simulink model "exploded_cbd"  (R2025b)
settings: Solver=VariableStepAuto  StartTime=0.0  StopTime=10.0  RelTol=1e-3
PreLoadFcn:
  | load 'Control Block Diagram'\contact_force.mat
model workspace (MAT data in the model file):
  B_imp = 1
  INA125_gain = 604
  J_imp = 1
  K_d = 1
  K_f = 1
  K_i = 1
  K_imp = 1
  K_p = 1
  finger_length = 0.105
  full_ROM = 90
  joint_pulley_diam = 0.1
  sine_freq_Hz = 2
libraries: simulink x3
settings Model: Creator=Madeline  LastModifiedBy=Madeline

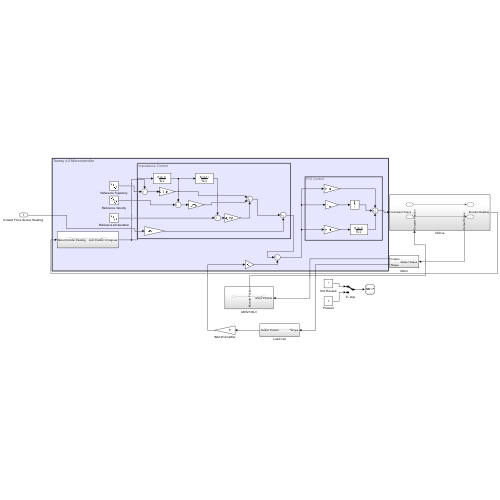
[thumbnail: Simulink's stored preview of the top-level diagram]
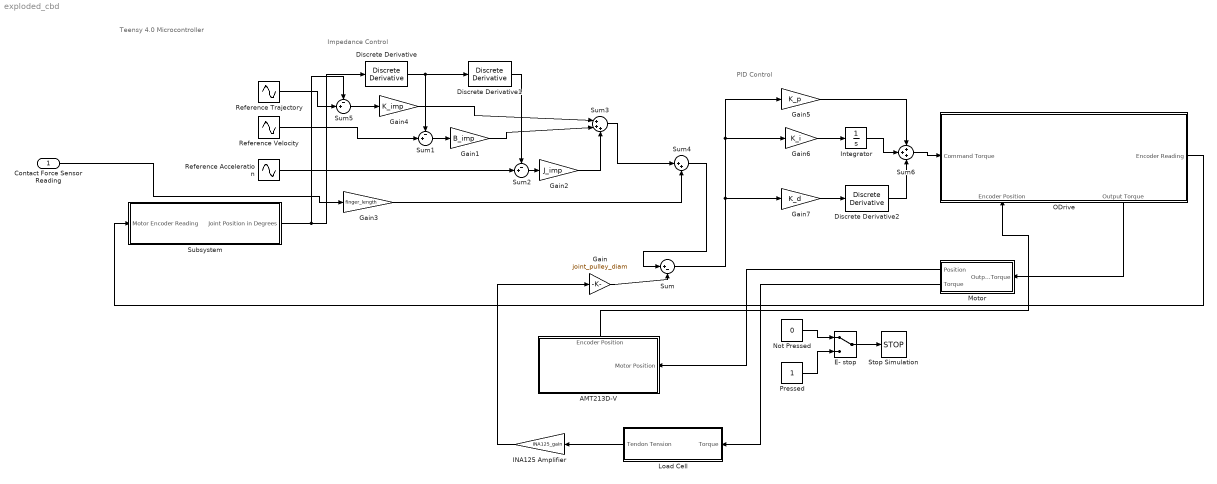
== system exploded_cbd ==
  note: PID Control
  note: Impedance Control
  note: Teensy 4.0 Microcontroller
  "Contact Force Sensor Reading " : Inport
  " E- stop" : ManualSwitch
  AMT213D-V : Subsystem
      settings: PortSchema="{\"entries\":[{\"content\":{\"sides\":[{\"content\":{\"connectorIds\":[\"In1\"]},\"type\":\"ConnectorPlacement.EquallySpacedRectSide\",\"uuid\":\"88afd67f-3209-48d2-80be-27a9c6027e98\"},{\"content\":{\"side\":\"RIGHT\"},\"type\":\"ConnectorPlacement.EquallySpacedRectSide\",\"uuid\":\"6bd83a64-80e2-4e6b-a2e1-60e2a1b1e7d1\"},{\"content\":{\"connectorIds\":[\"Out1\"],\"side\":\"TOP\"},\"type\":\"ConnectorPlacement.EquallySpacedRectSide\",\"uuid\":\"ca5e5761-7c4c-4ffd-94f8-cf864c9b5854\"}]},\"type\":\"ConnectorPlacement.EquallySpacedConnector\",\"uuid\":\"578619f2-0797-4ece-88f8-3f0e3f24fe58\"}],\"packageUris\":[\"http://schema.mathworks.com/mf0/Connector/R2020b\"],\"version\":\"1.0\"}"
  Discrete Derivative : simulink/Discrete/Discrete Derivative  gainval=1.0  ICPrevScaledInput=0.0  OutMin=[]  OutMax=[]  OutDataType=fixdt(1, 16)  OutScaling=2^-10  DoSatur=off
  Discrete Derivative1 : simulink/Discrete/Discrete Derivative  gainval=1.0  ICPrevScaledInput=0.0  OutMin=[]  OutMax=[]  OutDataType=fixdt(1, 16)  OutScaling=2^-10  DoSatur=off
  Discrete Derivative2 : simulink/Discrete/Discrete Derivative  gainval=1.0  ICPrevScaledInput=0.0  OutMin=[]  OutMax=[]  OutDataType=fixdt(1, 16)  OutScaling=2^-10  DoSatur=off
  Gain : Gain  Gain=joint_pulley_diam
  Gain1 : Gain  Gain=B_imp
  Gain2 : Gain  Gain=J_imp
  Gain3 : Gain  Gain=finger_length
  Gain4 : Gain  Gain=K_imp
  Gain5 : Gain  Gain=K_p
  Gain6 : Gain  Gain=K_i
  Gain7 : Gain  Gain=K_d
  INA125 Amplifier : Gain  Gain=INA125_gain
  Integrator : Integrator
  Load Cell : Subsystem
  Motor : Subsystem
  Not Pressed : Constant  Value=0
  ODrive : Subsystem
      settings: PortSchema="{\"entries\":[{\"content\":{\"sides\":[{\"content\":{\"connectorIds\":[\"In1\"]},\"type\":\"ConnectorPlacement.EquallySpacedRectSide\",\"uuid\":\"c97f3b25-cb08-4b77-804d-5691f1a52caa\"},{\"content\":{\"connectorIds\":[\"Out1\"],\"side\":\"RIGHT\"},\"type\":\"ConnectorPlacement.EquallySpacedRectSide\",\"uuid\":\"fc8ddf87-a458-4f73-a642-c7dd3d8cebff\"},{\"content\":{\"side\":\"TOP\"},\"type\":\"ConnectorPlacement.EquallySpacedRectSide\",\"uuid\":\"bec86457-f3cb-49fd-a085-c16f63c32d9e\"},{\"content\":{\"connectorIds\":[\"In2\",\"Out2\"],\"side\":\"BOTTOM\"},\"type\":\"ConnectorPlacement.EquallySpacedRectSide\",\"uuid\":\"4c0a5cbf-4f1d-4d43-a541-d1307432e3c9\"}]},\"type\":\"ConnectorPlacement.EquallySpacedConnector\",\"uuid\":\"94b3d347-19f8-405c-b5ff-c5a65504f3eb\"}],\"packageUris\":[\"http://schema.mathworks.com/mf0/Connector/R2020b\"],\"version\":\"1.0\"}"
  Pressed : Constant
  Reference Acceleration : Sin  Amplitude=-0.75*full_ROM*(sine_freq_Hz*2*pi)^2  Frequency=sine_freq_Hz*2*pi  SampleTime=0
  Reference Trajectory : Sin  Amplitude=0.75*full_ROM  Frequency=sine_freq_Hz*2*pi  SampleTime=0
  Reference Velocity : Sin  Amplitude=0.75*full_ROM*sine_freq_Hz*2*pi  Frequency=sine_freq_Hz*2*pi  Phase=pi/2  SampleTime=0
  Stop Simulation : Stop
  Subsystem : Subsystem
  Sum : Sum  Inputs=|+-
  Sum1 : Sum  Inputs=-+|
  Sum2 : Sum  Inputs=-+|
  Sum3 : Sum  Inputs=|+++
  Sum4 : Sum  Inputs=|++
  Sum5 : Sum  Inputs=-+|
  Sum6 : Sum  Inputs=+++
  wires:
  ODrive/2("Output Torque ") -> Motor/1("Output Torque ")
  Motor/1("Position ") -> AMT213D-V/1(Motor Position)
  Sum6/1 -> ODrive/1(Command Torque)
  AMT213D-V/1(Encoder Position) -> ODrive/2(Encoder Position)
  Motor/2(Torque) -> Load Cell/1(Torque)
  Not Pressed/1 -> " E- stop"/1
  Pressed/1 -> " E- stop"/2
  " E- stop"/1 -> Stop Simulation/1
  Load Cell/1(Tendon Tension) -> INA125 Amplifier/1
  Gain/1 -> Sum/2
  INA125 Amplifier/1 -> Gain/1
  Sum4/1 -> Sum/1
  ODrive/1(Encoder Reading) -> Subsystem/1(Motor Encoder Reading)
  Sum3/1 -> Sum4/1
  Gain3/1 -> Sum4/2
  "Contact Force Sensor Reading "/1 -> Gain3/1
  Gain2/1 -> Sum3/3
  Gain1/1 -> Sum3/2
  Gain4/1 -> Sum3/1
  Sum2/1 -> Gain2/1
  Sum1/1 -> Gain1/1
  Sum5/1 -> Gain4/1
  Reference Acceleration/1 -> Sum2/2
  Discrete Derivative1/1 -> Sum2/1
  Reference Velocity/1 -> Sum1/2
  Discrete Derivative/1 -> Sum1/1, Discrete Derivative1/1
  Subsystem/1(Joint Position in Degrees) -> Sum5/1, Discrete Derivative/1
  Reference Trajectory/1 -> Sum5/2
  Discrete Derivative2/1 -> Sum6/3
  Integrator/1 -> Sum6/2
  Gain5/1 -> Sum6/1
  Gain6/1 -> Integrator/1
  Gain7/1 -> Discrete Derivative2/1
  Sum/1 -> Gain5/1, Gain6/1, Gain7/1

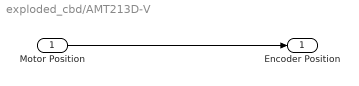
== system exploded_cbd/AMT213D-V ==
  Motor Position : Inport
  Encoder Position : Outport
  wires:
  Motor Position/1 -> Encoder Position/1

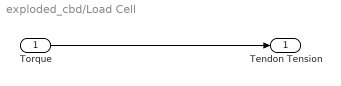
== system exploded_cbd/Load Cell ==
  Torque : Inport
  Tendon Tension : Outport
  wires:
  Torque/1 -> Tendon Tension/1

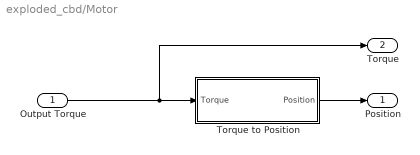
== system exploded_cbd/Motor ==
  "Output Torque " : Inport
  Torque to Position : Subsystem
  "Position " : Outport
  Torque : Outport  Port=2
  wires:
  Torque to Position/1(Position) -> "Position "/1
  "Output Torque "/1 -> Torque to Position/1("Torque "), Torque/1

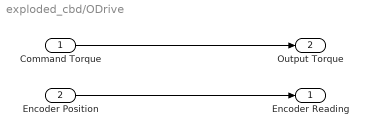
== system exploded_cbd/ODrive ==
  Command Torque : Inport
  Encoder Position : Inport  Port=2
  Encoder Reading : Outport
  "Output Torque " : Outport  Port=2
  wires:
  Command Torque/1 -> "Output Torque "/1
  Encoder Position/1 -> Encoder Reading/1

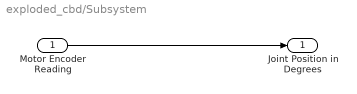
== system exploded_cbd/Subsystem ==
  Motor Encoder Reading : Inport
  Joint Position in Degrees : Outport
  wires:
  Motor Encoder Reading/1 -> Joint Position in Degrees/1

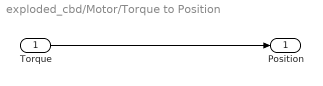
== system exploded_cbd/Motor/Torque to Position ==
  "Torque " : Inport
  Position : Outport
  wires:
  "Torque "/1 -> Position/1
